simulink model "LATC_Test_Calc"  (R2021b)
settings: Solver=FixedStepDiscrete  StartTime=0.0  StopTime=inf  FixedStep=0.01  RelTol=1e-3
values from neighbouring files (symbols this model uses):
  P_Global_CharSpd_ms : value not decoded    [PubParsGlobal.sldd]
  P_Global_SteeringAngleRatio : value not decoded    [PubParsGlobal.sldd]
  P_Global_WheelBase_m : value not decoded    [PubParsGlobal.sldd]
  P_LCS_A0_Dis_BP : value not decoded    [SubMdlDD_LATC.sldd]
  P_LCS_A2_Curve_BP : value not decoded    [SubMdlDD_LATC.sldd]
  P_LCS_A2_LatAcc_BP : value not decoded    [SubMdlDD_LATC.sldd]
  P_LCS_A2_Pretime = 0.075    [SubMdlDD_LATC.sldd]
  P_LCS_A2S_FliterTime = 0.5    [SubMdlDD_LATC.sldd]
  P_LCS_AngleFilterTime = 0.1    [SubMdlDD_LATC.sldd]
  P_LCS_AngleSlope_AES_Active = 0.4 0.4 0.4 0.35 0.35 0.35 0.35 0.35 0.35 0.3 0.3 0.3 0.3 0.3 0.3 0.3 0.3 0.3 0.3 0.4 0.4 0.4 0.35 0.35 0.35 0.35 0.35 0.35 0.3 0.3 0.3 0.3 0.3 0.3 0.3 0.3 0.3 0.3 0.4 0.4 0.4 0.35 0.35 0.35 0.35 0.35 0.35 0.3 0.3 0.3 0.3 0.3 0.3 0.3 0.3 0.3 0.3 0.4 0.4 0.4 0.35 0.35 0.35 0.35 0.35 0.35 0.3 0.3 0.3 0.3 0.3 0.3 0.3 0.3 0.3 0.3 0.4 0.4 0.4 0.35 0.35 0.35 0.35 0.35 0.35 0.3 0.3 0.3 0.3 0.3 0.3 0.3 0.    [SubMdlDD_LATC.sldd]
  P_LCS_AngleSlope_ESS_Add = 1.0 1.0 1.0 1.0 2.0 2.0 2.0 7.0 7.0 7.0 7.0 7.0 7.0 7.0 7.0 7.0 7.0 7.0 7.0 1.0 1.0 1.0 1.0 2.0 2.0 2.0 7.0 7.0 7.0 7.0 7.0 7.0 7.0 7.0 7.0 7.0 7.0 7.0 1.0 1.0 1.0 1.0 2.0 2.0 2.0 7.0 7.0 7.0 7.0 7.0 7.0 7.0 7.0 7.0 7.0 7.0 7.0 1.0 1.0 1.0 1.0 2.0 2.0 2.0 7.0 7.0 7.0 7.0 7.0 7.0 7.0 7.0 7.0 7.0 7.0 7.0 1.0 1.0 1.0 1.0 7.5 7.5 7.5 7.5 7.5 7.5 7.5 7.5 7.5 7.5 7.5 8.0 8.0 8.0 8.0 1.0 1.0 1.0 1.0 7.5    [SubMdlDD_LATC.sldd]
  P_LCS_AngleSlope_LC_Eco = 0.4 0.4 0.4 0.35 0.35 0.35 0.35 0.35 0.35 0.3 0.3 0.3 0.3 0.3 0.3 0.3 0.3 0.3 0.3 0.4 0.4 0.4 0.35 0.35 0.35 0.35 0.35 0.35 0.3 0.3 0.3 0.3 0.3 0.3 0.3 0.3 0.3 0.3 0.4 0.4 0.4 0.35 0.35 0.35 0.35 0.35 0.35 0.3 0.3 0.3 0.3 0.3 0.3 0.3 0.3 0.3 0.3 0.4 0.4 0.4 0.35 0.35 0.35 0.35 0.35 0.35 0.3 0.3 0.3 0.3 0.3 0.3 0.3 0.3 0.3 0.3 0.4 0.4 0.4 0.35 0.35 0.35 0.35 0.35 0.35 0.3 0.3 0.3 0.3 0.3 0.3 0.3 0.    [SubMdlDD_LATC.sldd]
  P_LCS_AngleSlope_LC_Nomal = 0.4 0.4 0.4 0.35 0.35 0.35 0.35 0.35 0.35 0.3 0.3 0.3 0.3 0.3 0.3 0.3 0.3 0.3 0.3 0.4 0.4 0.4 0.35 0.35 0.35 0.35 0.35 0.35 0.3 0.3 0.3 0.3 0.3 0.3 0.3 0.3 0.3 0.3 0.4 0.4 0.4 0.35 0.35 0.35 0.35 0.35 0.35 0.3 0.3 0.3 0.3 0.3 0.3 0.3 0.3 0.3 0.3 0.4 0.4 0.4 0.35 0.35 0.35 0.35 0.35 0.35 0.3 0.3 0.3 0.3 0.3 0.3 0.3 0.3 0.3 0.3 0.4 0.4 0.4 0.35 0.35 0.35 0.35 0.35 0.35 0.3 0.3 0.3 0.3 0.3 0.3 0.3 0.    [SubMdlDD_LATC.sldd]
  P_LCS_AngleSlope_LC_Sport = 0.4 0.4 0.4 0.35 0.35 0.35 0.35 0.35 0.35 0.3 0.3 0.3 0.3 0.3 0.3 0.3 0.3 0.3 0.3 0.4 0.4 0.4 0.35 0.35 0.35 0.35 0.35 0.35 0.3 0.3 0.3 0.3 0.3 0.3 0.3 0.3 0.3 0.3 0.4 0.4 0.4 0.35 0.35 0.35 0.35 0.35 0.35 0.3 0.3 0.3 0.3 0.3 0.3 0.3 0.3 0.3 0.3 0.4 0.4 0.4 0.35 0.35 0.35 0.35 0.35 0.35 0.3 0.3 0.3 0.3 0.3 0.3 0.3 0.3 0.3 0.3 0.4 0.4 0.4 0.35 0.35 0.35 0.35 0.35 0.35 0.3 0.3 0.3 0.3 0.3 0.3 0.3 0.    [SubMdlDD_LATC.sldd]
  P_LCS_AngleSlope_LCK = 0.4 0.4 0.4 0.4 0.4 0.4 0.4 0.4 0.4 0.4 0.4 0.4 0.4 0.4 0.4 0.4 0.4 0.4 0.4 0.4 0.4 0.4 0.4 0.4 0.4 0.4 0.4 0.4 0.4 0.4 0.4 0.4 0.4 0.4 0.4 0.4 0.4 0.4 0.4 0.4 0.4 0.4 0.4 0.4 0.4 0.4 0.4 0.4 0.4 0.4 0.4 0.4 0.4 0.4 0.4 0.4 0.4 0.4 0.4 0.4 0.4 0.4 0.4 0.4 0.4 0.4 0.4 0.4 0.4 0.4 0.4 0.4 0.4 0.4 0.4 0.4 0.4 0.4 0.4 0.4 0.4 0.4 0.4 0.4 0.4 0.4 0.4 0.4 0.4 0.4 0.4 0.4 0.4 0.4 0.4 0.4 0.4 0.4 0.4 0.4    [SubMdlDD_LATC.sldd]
  P_LCS_AngleSlope_LCKIE = 0.4 0.4 0.4 0.4 0.4 0.4 0.4 0.4 0.4 0.4 0.4 0.4 0.4 0.4 0.4 0.4 0.4 0.4 0.4 0.4 0.4 0.4 0.4 0.4 0.4 0.4 0.4 0.4 0.4 0.4 0.4 0.4 0.4 0.4 0.4 0.4 0.4 0.4 0.4 0.4 0.4 0.4 0.4 0.4 0.4 0.4 0.4 0.4 0.4 0.4 0.4 0.4 0.4 0.4 0.4 0.4 0.4 0.4 0.4 0.4 0.4 0.4 0.4 0.4 0.4 0.4 0.4 0.4 0.4 0.4 0.4 0.4 0.4 0.4 0.4 0.4 0.4 0.4 0.4 0.4 0.4 0.4 0.4 0.4 0.4 0.4 0.4 0.4 0.4 0.4 0.4 0.4 0.4 0.4 0.4 0.4 0.4 0.4 0.4 0.4    [SubMdlDD_LATC.sldd]
  P_LCS_AngleSlope_LKA = 0.2 0.2 0.3 0.4 0.4 0.4 0.4 0.4 0.4 0.4 0.4 0.4 0.4 0.4 0.4 0.4 0.4 0.4 0.4 0.2 0.2 0.3 0.4 0.4 0.4 0.4 0.4 0.4 0.4 0.4 0.4 0.4 0.4 0.4 0.4 0.4 0.4 0.4 0.2 0.2 0.3 0.4 0.4 0.4 0.4 0.4 0.4 0.4 0.4 0.4 0.4 0.4 0.4 0.4 0.4 0.4 0.4 0.2 0.2 0.3 0.4 0.4 0.4 0.4 0.4 0.4 0.4 0.4 0.4 0.4 0.4 0.4 0.4 0.4 0.4 0.4 0.2 0.2 0.3 0.4 0.4 0.4 0.4 0.4 0.4 0.4 0.4 0.4 0.4 0.4 0.4 0.4 0.4 0.4 0.4 0.2 0.2 0.3 0.4 0.4    [SubMdlDD_LATC.sldd]
  P_LCS_AngleSlope_Spd_BP : value not decoded    [SubMdlDD_LATC.sldd]
  P_LCS_DeltaEps_SpdBp : value not decoded    [SubMdlDD_LATC.sldd]
  P_LCS_DeltaEps_TimeVal : value not decoded    [SubMdlDD_LATC.sldd]
  P_LCS_DetNoOverRide_DrvTrq_TH : value not decoded    [SubMdlDD_LATC.sldd]
  P_LCS_DetOverRide_DrvTrq_TH : value not decoded    [SubMdlDD_LATC.sldd]
  P_LCS_ESS_AngleSlope_Limit = 2.9    [SubMdlDD_LATC.sldd]
  P_LCS_ESSAngleSW2 = 0.0    [SubMdlDD_LATC.sldd]
  P_LCS_LatAcc2CurveSW = 0.0    [SubMdlDD_LATC.sldd]
  P_LCS_LC_Complete_PreDisFac : value not decoded    [SubMdlDD_LATC.sldd]
  P_LCS_LCK_preDis_Nomal : value not decoded    [SubMdlDD_LATC.sldd]
  P_LCS_NoOverRideTime_TH_s : value not decoded    [SubMdlDD_LATC.sldd]
  P_LCS_OverRideDetect_enable : value not decoded    [SubMdlDD_LATC.sldd]
  P_LCS_OverRideTime_TH_s : value not decoded    [SubMdlDD_LATC.sldd]
  P_LCS_preDis_AES_Fac = 0.0 0.0 0.0 0.0 -0.1 -0.1 -0.1 -0.1 -0.1 -0.1 0.1 0.1 0.1 0.2 0.2 0.2 0.2 0.2 0.2 0.0 0.0 0.0 0.0 -0.1 -0.1 -0.1 -0.1 -0.1 -0.1 0.1 0.1 0.1 0.2 0.2 0.2 0.2 0.2 0.2 0.0 0.0 0.0 0.0 -0.1 -0.1 -0.1 -0.1 -0.1 -0.1 0.1 0.1 0.1 0.2 0.2 0.2 0.2 0.2 0.2 0.0 0.0 0.0 0.0 -0.1 -0.1 -0.1 -0.1 -0.1 -0.1 0.1 0.1 0.1 0.2 0.2 0.2 0.2 0.2 0.2 0.0 0.0 0.0 0.0 -0.1 -0.1 -0.1 -0.1 -0.1 -0.1 0.2 0.2 0.2 0.35 0.35 0.35    [SubMdlDD_LATC.sldd]
  P_LCS_preDis_LC_Eco_Fac = 0.0 0.0 0.0 0.0 0.25 0.3 0.3 0.3 0.35 0.35 0.45 0.45 0.45 0.55 0.55 0.55 0.55 0.55 0.55 0.0 0.0 0.0 0.0 0.25 0.3 0.3 0.3 0.35 0.35 0.45 0.45 0.45 0.55 0.55 0.55 0.55 0.55 0.55 0.0 0.0 0.0 0.0 0.25 0.3 0.3 0.3 0.35 0.35 0.45 0.45 0.45 0.55 0.55 0.55 0.55 0.55 0.55 0.0 0.0 0.0 0.0 0.25 0.3 0.3 0.3 0.35 0.35 0.45 0.45 0.45 0.55 0.55 0.55 0.55 0.55 0.55 0.0 0.0 0.0 0.0 0.25 0.3 0.3 0.3 0.35 0.35 0.55    [SubMdlDD_LATC.sldd]
  P_LCS_preDis_LC_Fac = 0.0 0.0 0.0 0.0 -0.1 -0.1 -0.1 -0.1 -0.1 -0.1 0.1 0.1 0.1 0.2 0.2 0.2 0.2 0.2 0.2 0.0 0.0 0.0 0.0 -0.1 -0.1 -0.1 -0.1 -0.1 -0.1 0.1 0.1 0.1 0.2 0.2 0.2 0.2 0.2 0.2 0.0 0.0 0.0 0.0 -0.1 -0.1 -0.1 -0.1 -0.1 -0.1 0.1 0.1 0.1 0.2 0.2 0.2 0.2 0.2 0.2 0.0 0.0 0.0 0.0 -0.1 -0.1 -0.1 -0.1 -0.1 -0.1 0.1 0.1 0.1 0.2 0.2 0.2 0.2 0.2 0.2 0.0 0.0 0.0 0.0 -0.1 -0.1 -0.1 -0.1 -0.1 -0.1 0.2 0.2 0.2 0.35 0.35 0.35    [SubMdlDD_LATC.sldd]
  P_LCS_preDis_LC_Nomal_Fac = 0.0 0.0 0.0 0.0 -0.1 -0.1 -0.1 -0.1 -0.1 -0.1 0.1 0.1 0.1 0.2 0.2 0.2 0.2 0.2 0.2 0.0 0.0 0.0 0.0 -0.1 -0.1 -0.1 -0.1 -0.1 -0.1 0.1 0.1 0.1 0.2 0.2 0.2 0.2 0.2 0.2 0.0 0.0 0.0 0.0 -0.1 -0.1 -0.1 -0.1 -0.1 -0.1 0.1 0.1 0.1 0.2 0.2 0.2 0.2 0.2 0.2 0.0 0.0 0.0 0.0 -0.1 -0.1 -0.1 -0.1 -0.1 -0.1 0.1 0.1 0.1 0.2 0.2 0.2 0.2 0.2 0.2 0.0 0.0 0.0 0.0 -0.1 -0.1 -0.1 -0.1 -0.1 -0.1 0.2 0.2 0.2 0.35 0.35 0.35    [SubMdlDD_LATC.sldd]
  P_LCS_preDis_LC_Sport_Fac = 0.0 0.0 0.0 0.0 -0.1 -0.1 -0.1 -0.1 -0.1 -0.1 0.1 0.1 0.1 0.2 0.2 0.2 0.2 0.2 0.2 0.0 0.0 0.0 0.0 -0.1 -0.1 -0.1 -0.1 -0.1 -0.1 0.1 0.1 0.1 0.2 0.2 0.2 0.2 0.2 0.2 0.0 0.0 0.0 0.0 -0.1 -0.1 -0.1 -0.1 -0.1 -0.1 0.1 0.1 0.1 0.2 0.2 0.2 0.2 0.2 0.2 0.0 0.0 0.0 0.0 -0.1 -0.1 -0.1 -0.1 -0.1 -0.1 0.1 0.1 0.1 0.2 0.2 0.2 0.2 0.2 0.2 0.0 0.0 0.0 0.0 -0.1 -0.1 -0.1 -0.1 -0.1 -0.1 0.2 0.2 0.2 0.35 0.35 0.35    [SubMdlDD_LATC.sldd]
  P_LCS_preDis_LCK_A2Curve_Fac2 : value not decoded    [SubMdlDD_LATC.sldd]
  P_LCS_preDis_spd : value not decoded    [SubMdlDD_LATC.sldd]
  P_LCS_StateActive_HoldTime_BP : value not decoded    [SubMdlDD_LATC.sldd]
  P_LCS_StateComplete_AngleSlope : value not decoded    [SubMdlDD_LATC.sldd]
  P_LCS_StateCompleteFlg_BP : value not decoded    [SubMdlDD_LATC.sldd]
  P_LCS_StateHold_time = 250.0    [SubMdlDD_LATC.sldd]
undefined symbols (not defined in the file or in its folder): P_LCS_AngleSlope_ELK, P_LCS_AngleSlope_ESS, P_LCS_AngleSlope_LC_Cancel, P_LCS_AngleSlope_LCK_Curve_Fac, P_LCS_ESS_preDis_Nomal, P_LCS_ESSAngleSW, P_LCS_ESSAngSlope_SW, P_LCS_preDis_ELK_Fac, P_LCS_preDis_ESS_Fac, P_LCS_preDis_LCK_A2Curve_Fac, P_LCS_preDis_LCK_Fac, P_LCS_StateActiv_AngleSlope, P_LCS_StateActiveFlg_BP
libraries: canapelib x26, simulink x7
(part 2 of 2)

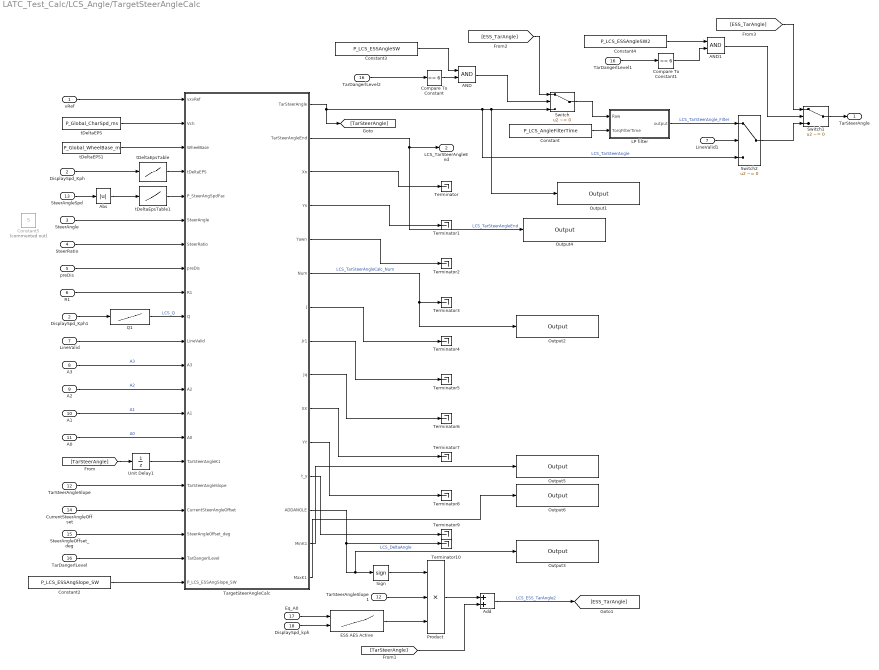
== system LATC_Test_Calc/LCS_Angle/TargetSteerAngleCalc ==
  vRef : Inport
  DisplaySpd_Kph : Inport  Port=2
  SteerAngle : Inport  Port=3
  SteerRatio : Inport  Port=4
  preDis : Inport  Port=5
  R1 : Inport  Port=6
  LineValid : Inport  Port=7
  A3 : Inport  Port=8
  A2 : Inport  Port=9
  A1 : Inport  Port=10
  A0 : Inport  Port=11
  "TarSteerAngleSlope " : Inport  Port=12
  SteerAngleSpd : Inport  Port=13
  CurrentSteerAngleOffset : Inport  Port=14
  SteerAngleOffset_deg : Inport  Port=15
  TarDangerlLevel : Inport  Port=16
  Eq_A0 : Inport  Port=17
  DisplaySpd_kph : Inport  Port=18
  AND : Logic  AllPortsSameDT=off  OutDataTypeStr=boolean
  AND1 : Logic  AllPortsSameDT=off  OutDataTypeStr=boolean
  Abs : Abs
  Add : Sum
  Compare To Constant : simulink/Logic and Bit Operations/Compare To Constant  relop===  const=6  OutDataTypeStr=boolean
  Compare To Constant1 : simulink/Logic and Bit Operations/Compare To Constant  relop===  const=6  OutDataTypeStr=boolean
  Constant : Constant  Value=P_LCS_AngleFilterTime
  Constant2 : Constant  Value=P_LCS_ESSAngSlope_SW
  Constant3 : Constant  Value=P_LCS_ESSAngleSW  OutDataTypeStr=boolean
  Constant4 : Constant  Value=P_LCS_ESSAngleSW2
  Constant5 : Constant  Commented=on  Value=5  OutDataTypeStr=single
  DisplaySpd_Kph1 : InportShadow  Port=2
  ESS AES Active : Lookup_n-D  BreakpointsForDimension1=P_LCS_A0_Dis_BP  BreakpointsForDimension2=P_LCS_AngleSlope_Spd_BP  Table=P_LCS_AngleSlope_ESS_Add  ExtrapMethod=Clip  UseLastTableValue=on  InternalRulePriority=Speed  OutDataTypeStr=single  RndMeth=Simplest
      settings: InputPortMap=u0,u1
  LP filter : Subsystem
  LineValid1 : InportShadow  Port=7
  Output1 : canapelib/CANape I//O/Output  envName=LCS_TarSteerAngle2  envRows=1  envCols=1  envPortId=0
      settings: AttributesFormatString=%<envName>  SourceProductName=Vector CANape/vSignalyzer Target
  Output2 : canapelib/CANape I//O/Output  envName=LCS_TarSteerAngleCalc_Num  envRows=1  envCols=1  envPortId=0
      settings: AttributesFormatString=%<envName>  SourceProductName=Vector CANape/vSignalyzer Target
  Output3 : canapelib/CANape I//O/Output  envName=LCS_DeltaAngle2  envRows=1  envCols=1  envPortId=0
      settings: AttributesFormatString=%<envName>  SourceProductName=Vector CANape/vSignalyzer Target
  Output4 : canapelib/CANape I//O/Output  envName=LCS_TarSteerAngleEnd2  envRows=1  envCols=1  envPortId=0
      settings: AttributesFormatString=%<envName>  SourceProductName=Vector CANape/vSignalyzer Target
  Output5 : canapelib/CANape I//O/Output  envName=MinK1  envRows=1  envCols=1  envPortId=0
      settings: AttributesFormatString=%<envName>  SourceProductName=Vector CANape/vSignalyzer Target
  Output6 : canapelib/CANape I//O/Output  envName=MaxK1  envRows=1  envCols=1  envPortId=0
      settings: AttributesFormatString=%<envName>  SourceProductName=Vector CANape/vSignalyzer Target
  Product : Product  Inputs=3  OutDataTypeStr=single
  Q1 : Lookup_n-D  NumberOfTableDimensions=1  BreakpointsForDimension1=[0,5,10,15,20,25,30,35,40,60,80,90,100,110,120,140]  Table=[0,0,0,0,0,0,0,0,0,0,0,0,0,0,0,0]  InternalRulePriority=Speed  RndMeth=Simplest  InputSameDT=on
  Sign : Signum
  Switch : Switch  Criteria=u2 ~= 0
  Switch1 : Switch  Criteria=u2 ~= 0
  Switch2 : Switch  Criteria=u2 ~= 0
  TarDangerlLevel1 : InportShadow  Port=16
  TarDangerlLevel2 : InportShadow  Port=16
  TarSteerAngleSlope 1 : InportShadow  Port=12
  TargetSteerAngleCalc : MATLAB Function  TreatAsAtomicUnit=on
  Terminator{,1..10} (11 alike) : Terminator
  Unit Delay1 : UnitDelay  SampleTime=-1  HasFrameUpgradeWarning=on
  tDeltaEPS : Constant  Value=P_Global_CharSpd_ms
  tDeltaEPS1 : Constant  Value=P_Global_WheelBase_m
  tDeltaEpsTable : Lookup_n-D  NumberOfTableDimensions=1  BreakpointsForDimension1=P_LCS_DeltaEps_SpdBp  Table=P_LCS_DeltaEps_TimeVal  ExtrapMethod=Clip  InternalRulePriority=Speed  RndMeth=Simplest  InputSameDT=on
  tDeltaEpsTable1 : Lookup_n-D  NumberOfTableDimensions=1  BreakpointsForDimension1=[0 10 20 30 50 100 200 300]  Table=[1 1 1 1 1 0.5 0.2 0.2]  ExtrapMethod=Clip  UseLastTableValue=on  InternalRulePriority=Speed  RndMeth=Simplest  InputSameDT=on
  TarSteerAngle : Outport
  LCS_TarSteerAngleEnd : Outport  Port=2
  wires:
  LineValid1/1 -> Switch2/2
  Switch2/1 -> Switch1/3
  ESS AES Active/1 -> Product/3
  DisplaySpd_kph/1 -> ESS AES Active/2
  Eq_A0/1 -> ESS AES Active/1
  TarDangerlLevel2/1 -> Compare To Constant/1
  TarDangerlLevel1/1 -> Compare To Constant1/1
  TargetSteerAngleCalc/13(ADDANGLE) -> Output3/1, Sign/1, Terminator10/1  "LCS_DeltaAngle"
  Sign/1 -> Product/1
  TarSteerAngleSlope 1/1 -> Product/2
  Product/1 -> Add/1
  [TarSteerAngle] -> Add/2
  Add/1 -> [ESS_TarAngle]  "LCS_ESS_TarAngle2"
  TargetSteerAngleCalc/1(TarSteerAngle) -> [TarSteerAngle], Output1/1, Switch/3, Switch2/3  "LCS_TarSteerAngle"
  Constant/1 -> LP filter/2(TorqFilterTime)
  LP filter/1(output) -> Switch2/1  "LCS_TarSteerAngle_Filter"
  Switch/1 -> LP filter/1(Raw)
  [ESS_TarAngle] -> Switch/1
  Constant3/1 -> AND/1
  Compare To Constant/1 -> AND/2
  AND/1 -> Switch/2
  AND1/1 -> Switch1/2
  Compare To Constant1/1 -> AND1/2
  Constant4/1 -> AND1/1
  [ESS_TarAngle] -> Switch1/1
  Switch1/1 -> TarSteerAngle/1
  Constant2/1 -> TargetSteerAngleCalc/21(P_LCS_ESSAngSlope_SW)
  TarDangerlLevel/1 -> TargetSteerAngleCalc/20(TarDangerlLevel)
  TargetSteerAngleCalc/12(t_y) -> Terminator9/1
  TargetSteerAngleCalc/2(TarSteerAngleEnd) -> Output4/1, LCS_TarSteerAngleEnd/1  "LCS_TarSteerAngleEnd"
  preDis/1 -> TargetSteerAngleCalc/8(preDis)
  "TarSteerAngleSlope "/1 -> TargetSteerAngleCalc/17(TarSteerAngleSlope)
  Unit Delay1/1 -> TargetSteerAngleCalc/16(TarSteerAngleK1)
  tDeltaEpsTable1/1 -> TargetSteerAngleCalc/5(P_SteerAngSpdFac)
  vRef/1 -> TargetSteerAngleCalc/1(vxvRef)
  TargetSteerAngleCalc/11(YY) -> Terminator8/1
  TargetSteerAngleCalc/10(XX) -> Terminator7/1
  R1/1 -> TargetSteerAngleCalc/9(R1)
  SteerAngleSpd/1 -> Abs/1
  TargetSteerAngleCalc/9(Jq) -> Terminator6/1
  TargetSteerAngleCalc/8(Jr1) -> Terminator5/1
  TargetSteerAngleCalc/7(J) -> Terminator4/1
  TargetSteerAngleCalc/6(Num) -> Output2/1, Terminator3/1  "LCS_TarSteerAngleCalc_Num"
  TargetSteerAngleCalc/5(Yawn) -> Terminator2/1
  TargetSteerAngleCalc/4(Yn) -> Terminator1/1
  TargetSteerAngleCalc/3(Xn) -> Terminator/1
  SteerRatio/1 -> TargetSteerAngleCalc/7(SteerRatio)
  tDeltaEpsTable/1 -> TargetSteerAngleCalc/4(tDeltaEPS)
  DisplaySpd_Kph/1 -> tDeltaEpsTable/1
  A3/1 -> TargetSteerAngleCalc/12(A3)  "A3"
  A1/1 -> TargetSteerAngleCalc/14(A1)  "A1"
  A0/1 -> TargetSteerAngleCalc/15(A0)  "A0"
  A2/1 -> TargetSteerAngleCalc/13(A2)  "A2"
  tDeltaEPS/1 -> TargetSteerAngleCalc/2(Vch)
  tDeltaEPS1/1 -> TargetSteerAngleCalc/3(WheelBase)
  Q1/1 -> TargetSteerAngleCalc/10(Q)  "LCS_Q"
  DisplaySpd_Kph1/1 -> Q1/1
  CurrentSteerAngleOffset/1 -> TargetSteerAngleCalc/18(CurrentSteerAngleOffset)
  LineValid/1 -> TargetSteerAngleCalc/11(LineValid)
  SteerAngleOffset_deg/1 -> TargetSteerAngleCalc/19(SteerAngleOffset_deg)
  TargetSteerAngleCalc/14(MinK1) -> Output5/1
  TargetSteerAngleCalc/15(MaxK1) -> Output6/1
  [TarSteerAngle] -> Unit Delay1/1
  SteerAngle/1 -> TargetSteerAngleCalc/6(SteerAngle)
  Abs/1 -> tDeltaEpsTable1/1

== system LATC_Test_Calc/LCS_Angle/AngSlopeCalc/Switch Case Action Subsystem ==
  Flg : Inport
  StateHoldTime : Inport  Port=2
  Action Port : ActionPort  ActionPortLabel=case [ 1 2 3 4 5 6 ]:
  LC_start_slope : Lookup_n-D  BreakpointsForDimension1=P_LCS_StateActiveFlg_BP  BreakpointsForDimension2=P_LCS_StateActive_HoldTime_BP  Table=P_LCS_StateActiv_AngleSlope  ExtrapMethod=Clip  UseLastTableValue=on  InternalRulePriority=Speed  OutDataTypeStr=single  RndMeth=Simplest
      settings: InputPortMap=u0,u1
  Out1 : Outport
  wires:
  StateHoldTime/1 -> LC_start_slope/2
  LC_start_slope/1 -> Out1/1
  Flg/1 -> LC_start_slope/1

== system LATC_Test_Calc/LCS_Angle/AngSlopeCalc/Switch Case Action Subsystem1 ==
  Action Port : ActionPort  ActionPortLabel=default:
  Constant : Constant  Value=100  OutDataTypeStr=single
  Out1 : Outport
  wires:
  Constant/1 -> Out1/1

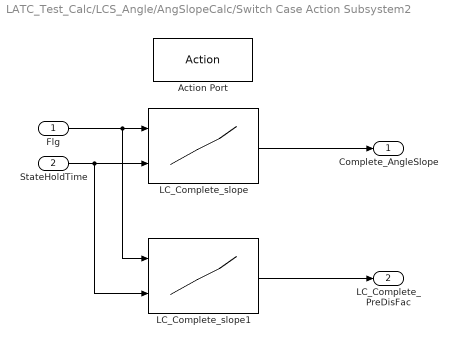
== system LATC_Test_Calc/LCS_Angle/AngSlopeCalc/Switch Case Action Subsystem2 ==
  Flg : Inport
  StateHoldTime : Inport  Port=2
  Action Port : ActionPort  ActionPortLabel=case [ 7 8 9 10 ]:
  LC_Complete_slope : Lookup_n-D  BreakpointsForDimension1=P_LCS_StateCompleteFlg_BP  BreakpointsForDimension2=P_LCS_StateActive_HoldTime_BP  Table=P_LCS_StateComplete_AngleSlope  ExtrapMethod=Clip  UseLastTableValue=on  InternalRulePriority=Speed  OutDataTypeStr=single  RndMeth=Simplest
      settings: InputPortMap=u0,u1
  LC_Complete_slope1 : Lookup_n-D  BreakpointsForDimension1=P_LCS_StateCompleteFlg_BP  BreakpointsForDimension2=P_LCS_StateActive_HoldTime_BP  Table=P_LCS_LC_Complete_PreDisFac  ExtrapMethod=Clip  UseLastTableValue=on  InternalRulePriority=Speed  OutDataTypeStr=single  RndMeth=Simplest
      settings: InputPortMap=u0,u1
  Complete_AngleSlope : Outport
  LC_Complete_PreDisFac : Outport  Port=2
  wires:
  LC_Complete_slope/1 -> Complete_AngleSlope/1
  Flg/1 -> LC_Complete_slope1/1, LC_Complete_slope/1
  StateHoldTime/1 -> LC_Complete_slope1/2, LC_Complete_slope/2
  LC_Complete_slope1/1 -> LC_Complete_PreDisFac/1

== system LATC_Test_Calc/LCS_Angle/AngSlopeCalc/Switch Case Action Subsystem3 ==
  Action Port : ActionPort  ActionPortLabel=default:
  Constant : Constant  Value=0.2  OutDataTypeStr=single
  Constant1 : Constant  OutDataTypeStr=single
  Complete_AngleSlope : Outport
  Complete_PreDisFac : Outport  Port=2
  wires:
  Constant/1 -> Complete_AngleSlope/1
  Constant1/1 -> Complete_PreDisFac/1

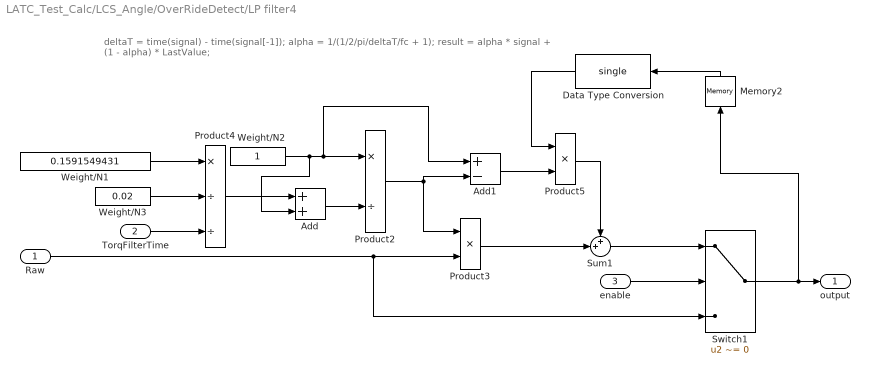
== system LATC_Test_Calc/LCS_Angle/OverRideDetect/LP filter4 ==
  note: deltaT = time(signal) - time(signal[-1]);
      |    alpha = 1/(1/2/pi/deltaT/fc + 1);
      |    result = alpha * signal + (1 - alpha) * LastValue;
  Raw : Inport
  TorqFilterTime : Inport  Port=2
  enable : Inport  Port=3
  Add : Sum
  Add1 : Sum  Inputs=+-
  Data Type Conversion : DataTypeConversion  OutDataTypeStr=single
  Memory2 : Memory  InheritSampleTime=on
  Product2 : Product  Inputs=*/  RndMeth=Zero
  Product3 : Product  RndMeth=Zero
  Product4 : Product  Inputs=*//  RndMeth=Zero
  Product5 : Product  RndMeth=Zero
  Sum1 : Sum  Inputs=++|
  Switch1 : Switch  Criteria=u2 ~= 0
  Weight/N1 : Constant  Value=0.1591549431  OutDataTypeStr=single
  Weight/N2 : Constant  OutDataTypeStr=single
  Weight/N3 : Constant  Value=0.02  OutDataTypeStr=single
  output : Outport
  wires:
  TorqFilterTime/1 -> Product4/3
  Product4/1 -> Add/1
  Weight/N3/1 -> Product4/2
  Memory2/1 -> Data Type Conversion/1
  enable/1 -> Switch1/2
  Raw/1 -> Product3/2, Switch1/3
  Switch1/1 -> output/1, Memory2/1
  Weight/N1/1 -> Product4/1
  Weight/N2/1 -> Add1/1, Product2/1, Add/2
  Add/1 -> Product2/2
  Product2/1 -> Product3/1, Add1/2
  Product3/1 -> Sum1/2
  Add1/1 -> Product5/2
  Product5/1 -> Sum1/1
  Sum1/1 -> Switch1/1
  Data Type Conversion/1 -> Product5/1

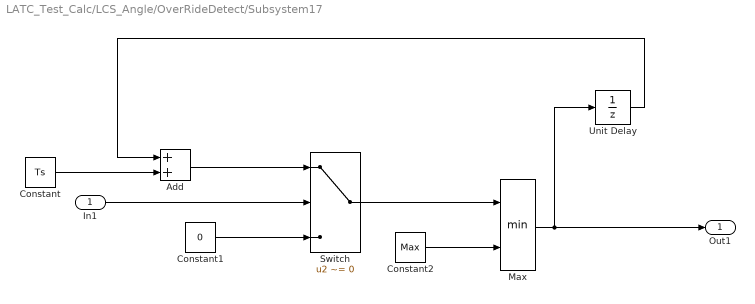
== system LATC_Test_Calc/LCS_Angle/OverRideDetect/Subsystem17 ==
  In1 : Inport
  Add : Sum
  Constant : Constant  Value=Ts
  Constant1 : Constant  Value=0
  Constant2 : Constant  Value=Max
  Max : MinMax  Inputs=2
  Switch : Switch  Criteria=u2 ~= 0
  Unit Delay : UnitDelay  SampleTime=-1  HasFrameUpgradeWarning=on
  Out1 : Outport
  wires:
  Switch/1 -> Max/1
  Constant2/1 -> Max/2
  Max/1 -> Out1/1, Unit Delay/1
  Add/1 -> Switch/1
  Constant1/1 -> Switch/3
  Constant/1 -> Add/2
  In1/1 -> Switch/2
  Unit Delay/1 -> Add/1

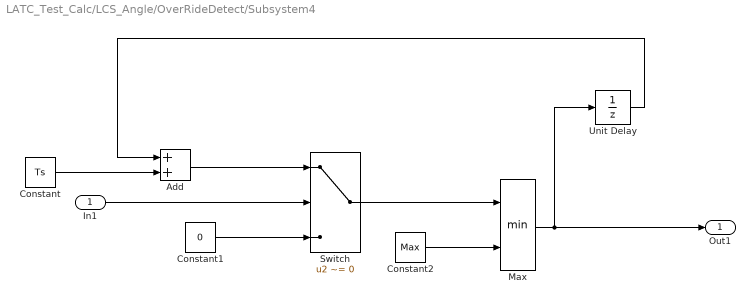
== system LATC_Test_Calc/LCS_Angle/OverRideDetect/Subsystem4 ==
  In1 : Inport
  Add : Sum
  Constant : Constant  Value=Ts
  Constant1 : Constant  Value=0
  Constant2 : Constant  Value=Max
  Max : MinMax  Inputs=2
  Switch : Switch  Criteria=u2 ~= 0
  Unit Delay : UnitDelay  SampleTime=-1  HasFrameUpgradeWarning=on
  Out1 : Outport
  wires:
  Unit Delay/1 -> Add/1
  In1/1 -> Switch/2
  Constant/1 -> Add/2
  Constant1/1 -> Switch/3
  Add/1 -> Switch/1
  Max/1 -> Unit Delay/1, Out1/1
  Constant2/1 -> Max/2
  Switch/1 -> Max/1

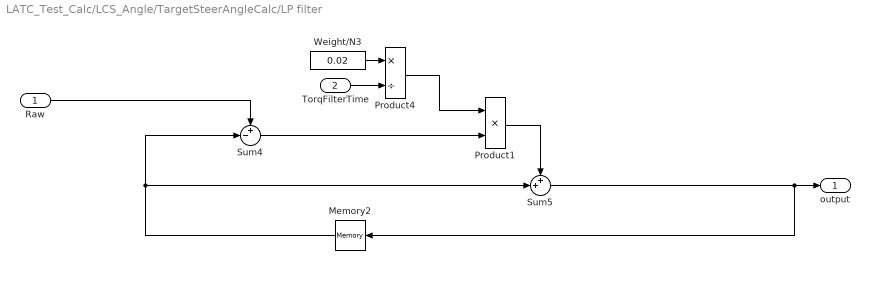
== system LATC_Test_Calc/LCS_Angle/TargetSteerAngleCalc/LP filter ==
  Raw : Inport
  TorqFilterTime : Inport  Port=2
  Memory2 : Memory  InheritSampleTime=on
  Product1 : Product  RndMeth=Zero
  Product4 : Product  Inputs=*/  RndMeth=Zero
  Sum4 : Sum  Inputs=+-|
  Sum5 : Sum  Inputs=++|
  Weight/N3 : Constant  Value=0.02  OutDataTypeStr=single
  output : Outport
  wires:
  Sum5/1 -> Memory2/1, output/1
  Memory2/1 -> Sum5/2, Sum4/2
  Sum4/1 -> Product1/2
  Product1/1 -> Sum5/1
  Raw/1 -> Sum4/1
  Weight/N3/1 -> Product4/1
  Product4/1 -> Product1/1
  TorqFilterTime/1 -> Product4/2

== matlab function LATC_Test_Calc/LCS_Angle/AngSlopeCalc/MATLAB Function3 ==
  data: delytime input uint16; TarDangerLevel input uint8; TarDangerLevelK1 input uint8; FLg output uint8; FLgK1 input uint8; CntK1 input uint16; Cnt output uint16
function [FLg,Cnt] = AngSlopeCalc(delytime,TarDangerLevel,TarDangerLevelK1,FLgK1,CntK1)

Cnt = min(CntK1 + uint16(1),delytime);
if Cnt== delytime
    FLg = uint8(0);
else
    FLg = FLgK1;
end
%FLg = FLgK1;
%% 
if TarDangerLevel==uint8(1) && TarDangerLevelK1==0  % NO function 2 LCK (TarDangerLevelK1==0)
    Cnt =uint16(0);
    FLg = uint8(1);
end

if  TarDangerLevel==uint8(3) && (TarDangerLevelK1==uint8(1)||TarDangerLevelK1==uint8(2)) % LCK/IE 2 LC_Normal
    Cnt =uint16(0);
    FLg = uint8(2);
end

if  TarDangerLevel==uint8(7) && (TarDangerLevelK1==uint8(1)||TarDangerLevelK1==uint8(2)) % LCK/IE 2 LC_Eco
    Cnt =uint16(0);
    FLg = uint8(3);
end

if  TarDangerLevel==uint8(8) && (TarDangerLevelK1==uint8(1)||TarDangerLevelK1==uint8(2)) % LCK/IE 2 LC_sport
    Cnt =uint16(0);
    FLg = uint8(4);
end
if  TarDangerLevel==uint8(6) && (TarDangerLevelK1==uint8(1)||TarDangerLevelK1==uint8(2)) % LCK/IE 2 ESS 后期添加配和ESS Slope 一起调试
    Cnt =uint16(0);
    FLg = uint8(5);
end
if  TarDangerLevel==uint8(10) && (TarDangerLevelK1==uint8(1)||TarDangerLevelK1==uint8(2)) % LCK/IE 2 AES 后期添加配和ESS Slope 一起调试
    Cnt =uint16(0);
    FLg = uint8(6);
end
%% 换道完成检测，主要时为了解决换道完成后切换到LCK后Angleslope太小导致超调，检测到换道完成后延时一段时间保持一个大斜率。
if  (TarDangerLevel==uint8(1)||TarDangerLevel==uint8(2)) && (TarDangerLevelK1==uint8(3)) % LCK/IE 2 LC_Normal Complete
    Cnt =uint16(0);
    FLg = uint8(7);
end
if  (TarDangerLevel==uint8(1)||TarDangerLevel==uint8(2)) && (TarDangerLevelK1==uint8(7)) % LCK/IE 2 LC_Eco Complete
    Cnt =uint16(0);
    FLg = uint8(8);
end
if  (TarDangerLevel==uint8(1)||TarDangerLevel==uint8(2)) && (TarDangerLevelK1==uint8(8)) % LCK/IE 2 LC_sport Complete
    Cnt =uint16(0);
    FLg = uint8(9);
end
if  (TarDangerLevel==uint8(1)||TarDangerLevel==uint8(2)) && (TarDangerLevelK1==uint8(10)) % LCK/IE 2 AES Complete
    Cnt =uint16(0);
    FLg = uint8(10);
end

== matlab function LATC_Test_Calc/LCS_Angle/MATLAB Function ==
  data: c2 input; c1 input; c3 input; v input; PreCurve output; time input
function PreCurve = fcn(c2,c1,c3,v,time)
pdis = v*time;
% y1 = 3*c3*pdis^2 + 2*c2*pdis + c1;
PreCurve = 6*c3*pdis + 2*c2;
% r = y2/power((1+y1*y1),single(1.5));
end

== stateflow chart LATC_Test_Calc/LCS_Angle/OverRideDetect/Chart ==
  state NoOverRide
    en:isOverRide=false;
  state IsOverRide
    en:isOverRide=true;
  (default) -> NoOverRide
  NoOverRide -> IsOverRide : [Ovride]
  IsOverRide -> NoOverRide : [NoOvride]
  data: isOverRide output; Ovride input; NoOvride input

== matlab function LATC_Test_Calc/LCS_Angle/TargetSteerAngleCalc/TargetSteerAngleCalc ==
  data: TarSteerAngle output single size=1; TarSteerAngleEnd output single size=1; Xn output single size=1; Yn output single size=1; Yawn output single size=1; Num output single size=1; J output single size=[31,1]; Jr1 output single size=[31,1]; Jq output single size=[31,1]; vxvRef input single size=1; Vch input single size=1; WheelBase input single size=1; tDeltaEPS input single size=1; P_SteerAngSpdFac input single size=1; SteerAngle input single size=1; SteerRatio input double size=1; preDis input single size=1; R1 input single size=1; Q input single size=1; LineValid input boolean size=1; A3 input single size=1; A2 input single size=1; A1 input single size=1; A0 input single size=1; TarSteerAngleK1 input single size=1; TarSteerAngleSlope input single size=1; XX output; YY output; t_y output; ADDANGLE output; CurrentSteerAngleOffset input single; SteerAngleOffset_deg input; TarDangerlLevel input; P_LCS_ESSAngSlope_SW input; MinK1 output; MaxK1 output
function [TarSteerAngle,TarSteerAngleEnd,Xn,Yn,Yawn,Num,J,Jr1,Jq,XX,YY,t_y,ADDANGLE,MinK1,MaxK1] = ...
    TargetSteerAngleCalc(vxvRef,Vch,WheelBase,tDeltaEPS,P_SteerAngSpdFac,SteerAngle,SteerRatio,preDis, R1,Q,...
    LineValid,A3,A2,A1,A0,TarSteerAngleK1,TarSteerAngleSlope,CurrentSteerAngleOffset,SteerAngleOffset_deg,TarDangerlLevel,P_LCS_ESSAngSlope_SW)

StrToWhlFac = 57.3*SteerRatio;
SteerAngleDt = single(TarSteerAngleSlope*50);
dxOffset = single(2.1);
J = single(zeros(31,1));
Jr1 = single(zeros(31,1));
Jq = single(zeros(31,1));
Num = single(0);
XX = single(zeros(1,20));
YY = single(zeros(1,20));
t_y = single(zeros(1,20));
ADDANGLE= 0;
MinK1 = single(zeros(1,1));
MaxK1 = single(zeros(1,1));
% deltaAngle = [-45.5, -34.4, -25.3, -18.0, -12.3, -8.0,...
%     -4.9, -2.8, -1.5, -0.8, -0.5, -0.4, -0.3, -0.2, -0.1, ...
%     0, 0.1, 0.2, 0.3, 0.4, 0.5, 0.8, 1.5, 2.8,...
%     4.9, 8.0, 12.3, 18.0, 25.3, 34.4, 45.5];
deltaAngle = [-8.0, -8.0, -8.0, -8.0, -8.0, -8.0,...
    -4.9, -2.8, -1.5, -0.8, -0.5, -0.4, -0.3, -0.2, -0.1, ...
    0, 0.1, 0.2, 0.3, 0.4, 0.5, 0.8, 1.5, 2.8,...
    4.9, 8.0, 8.0, 8.0, 8.0, 8.0, 8.0];

vRef = max(vxvRef,single(0.1));

if LineValid
    % 20 Calculate Cycle
    disStep = preDis/single(49);
    SteerAngleMa = single(zeros(31,20));
    YawMa = single(zeros(31,20));
    YiMa = single(zeros(31,20));
    XiMa = single(zeros(31,20));
    yValid = true(31,1);
    Jmin =single(-1);
    Num = single(0);
    
    for k=single(1:31)
        SteerAngleRaw = SteerAngle + deltaAngle(k); 
        % SteerAngleRaw = TarSteerAngleK1 + deltaAngle(k);
        tD = disStep/vRef; 
        
       
        %% 
        SteerAngleMa(k,1) =  TarSteerAngleK1;
        % SteerAngleMa(k,1) =  SteerAngle;
        for i=2:20
            if i<=5
                tDelta = tD;
            elseif i<=10
                tDelta = 2*tD;
            elseif i<=15
                tDelta = 3*tD;
            else
                tDelta = 4*tD;
            end
            % SteerAngleRaw>SteerAngle
            if SteerAngleRaw>SteerAngle
                SteerAngleMa(k,i) = SteerAngleMa(k,1) + tDelta*single((i-1))*SteerAngleDt;%
                SteerAngleMa(k,i) = min(SteerAngleMa(k,i),SteerAngleRaw);% 
            else
                SteerAngleMa(k,i) = SteerAngleMa(k,1) - tDelta*(single(i-1))*SteerAngleDt;
                SteerAngleMa(k,i) = max(SteerAngleMa(k,i),SteerAngleRaw);
            end
        end
        %% 
        % 
        if vRef<1
            YawMa(k,1) = tDeltaEPS*vRef*tan(P_SteerAngSpdFac*0.5*(SteerAngle + TarSteerAngleK1)/StrToWhlFac)/WheelBase; % 
        else
            AckConst = min((single(1)+vRef*vRef/(Vch*Vch))*WheelBase/max(single(1),vRef),single(32767));
            YawMa(k,1) =P_SteerAngSpdFac*0.5*tDeltaEPS*(SteerAngle + TarSteerAngleK1)/(AckConst*StrToWhlFac);
        end
        XiMa(k,1) = tDeltaEPS*vRef*cos(YawMa(k,1));%推算第一步纵向坐标
        YiMa(k,1) = tDeltaEPS*vRef*sin(YawMa(k,1));%推算第一步横向坐标
        %% 
        uDelta = SteerAngleRaw - SteerAngle;

        t_Start =single(18);
        t_End = single(19); 
        for i=1:t_End
            if i<=5
                disStepFac = single(1);
            elseif i<=10
                disStepFac = single(2);
            elseif i<=15
                disStepFac = single(3);
            else
                disStepFac = single(4);
            end
            if vRef<1
                t_kap = tan(SteerAngleMa(k,i)/StrToWhlFac)/WheelBase;
                YawMa(k,i+1) = YawMa(k,i) + disStepFac*disStep*t_kap;
            else
                tStep = disStepFac*disStep/vRef;
                AckConst = min((single(1)+vRef*vRef/(Vch*Vch))*WheelBase/vRef,single(32767));
                YawRate = SteerAngleMa(k,i)/(AckConst*StrToWhlFac);
                YawMa(k,i+1) = YawMa(k,i) + YawRate*tStep;
            end
            
            if (YawMa(k,i+1)>single(1.2))||(YawMa(k,i+1)<single(-1.2)) %
                yValid(k) = false;
            else
                XiMa(k,i+1) = XiMa(k,i) + disStepFac*disStep*cos(0.5*(YawMa(k,i)+YawMa(k,i+1)));
                YiMa(k,i+1) = YiMa(k,i) + disStepFac*disStep*sin(0.5*(YawMa(k,i)+YawMa(k,i+1)));
                
                if (i>t_Start)&&(i<=t_End)
                    t = XiMa(k,i+1) + dxOffset*cos(YawMa(k,i+1));
                    dy = YiMa(k,i+1) + dxOffset*sin(YawMa(k,i+1));
                    dyRef = A3*t^3 + A2*t^2 + A1*t + A0;
                    %AngleRef = atan(3*A3*dx^2 + 2*A2*dx + A1);
                    
                    Jr1(k) = R1*(dy - dyRef)^2;
                    J(k) = J(k) + Jr1(k);
                end
            end
        end
        %% 第K步的损失量
        Jq(k) = Q*uDelta^2;
        J(k) = J(k) + Jq(k);
        
        if (yValid(k)==true)
            if Jmin<0
                Jmin = J(k);
                Num = k;
            else
                if k<=16
                    if J(k)<=Jmin
                        Jmin = J(k);
                        Num = k;
                    end
                else
                    if J(k)<Jmin
                        Jmin = J(k);
                        Num = k;
                    end
                end
            end
        end
        
    end
    
    TarSteerAngleEnd = SteerAngle + deltaAngle(Num); 
    if TarDangerlLevel==6 && P_LCS_ESSAngSlope_SW ==1
        TarSteerAngle = min(SteerAngle + TarSteerAngleSlope,max(SteerAngle - TarSteerAngleSlope,TarSteerAngleEnd));
    else
        MinK1 = TarSteerAngleK1 - TarSteerAngleSlope;
        MaxK1 = TarSteerAngleK1 + TarSteerAngleSlope;
        TarSteerAngle = min(TarSteerAngleK1 + TarSteerAngleSlope,max(TarSteerAngleK1 - TarSteerAngleSlope,TarSteerAngleEnd));
    end
   
    Xn = XiMa(Num,t_End);
    Yn = YiMa(Num,t_End);
    Yawn = YawMa(Num,t_End);
    XX =  XiMa(Num,:);
    YY =  YiMa(Num,:);    
    for i = 1:20
        t_x = XiMa(Num,i);
        t_y(i) = A3*t_x^3 + A2*t_x^2 + A1*t_x + A0;
    end
    ADDANGLE=deltaAngle(Num);
else
    TarSteerAngle = SteerAngle+SteerAngleOffset_deg-CurrentSteerAngleOffset;
    TarSteerAngleEnd = SteerAngle;
    Xn = single(0);
    Yn = single(0);
    Yawn = single(0);
end
end
